simulink model "PID_nova_metoda"  (R2018a)
settings: Solver=ode4  StartTime=0.0  StopTime=100000.0  FixedStep=0.1  RelTol=1e-3
values from neighbouring files (symbols this model uses):
  Ca = pom1*10^-6    [projekat1.m]
  Cb = 10^-6    (= 1e-06)    [projekat1.m]
  Fa = 0.016667    [projekat1.m]
  Kp = mi*T*du/dy/tau    [projekat1.m]
  kw = 10^-14    (= 1e-14)    [projekat1.m]
  Td = T/8    [projekat1.m]
  Tf = Td/20    [projekat1.m]
  Ti = T    [projekat1.m]
  Tt = 0.01*Ti    (= 9.0009)    [projekat1.m]
  uep = eval (ue)    [projekat1.m]
  V = 30    [projekat1.m]
settings Model: Creator=Dusan Licina  LastModifiedBy=svorc

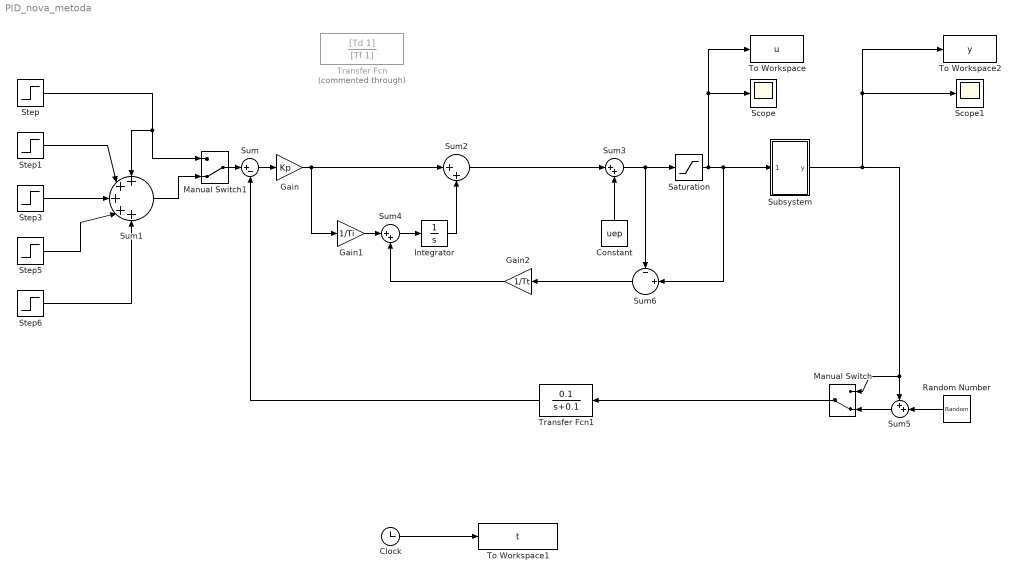
== system PID_nova_metoda ==
  Clock : Clock
  Constant : Constant  Value=uep
  Gain : Gain  Gain=Kp
  Gain1 : Gain  Gain=1/Ti
  Gain2 : Gain  Gain=1/Tt
  Integrator : Integrator
  Manual Switch : ManualSwitch  CurrentSetting=0
  Manual Switch1 : ManualSwitch  CurrentSetting=0
  Random Number : RandomNumber  Variance=0.1225  SampleTime=0.1
  Saturation : Saturate  UpperLimit=10*Fa  LowerLimit=0
  Scope : Scope
  Scope1 : Scope
  Step : Step  Time=0.1  After=7  SampleTime=0
  Step1 : Step  Time=10000  After=-0.5  SampleTime=0
  Step3 : Step  Time=30000  After=0.5  SampleTime=0
  Step5 : Step  Time=50000  After=0.5  SampleTime=0
  Step6 : Step  Time=70000  After=-0.5  SampleTime=0
  Subsystem : Subsystem
  Sum : Sum  Inputs=|+-
  Sum1 : Sum  Inputs=+|+|+|+|+
  Sum2 : Sum  Inputs=|++
  Sum3 : Sum  Inputs=|++
  Sum4 : Sum  Inputs=|++
  Sum5 : Sum  Inputs=++|
  Sum6 : Sum  Inputs=-|+||
  To Workspace : ToWorkspace  VariableName=u  SampleTime=-1
  To Workspace1 : ToWorkspace  VariableName=t  SampleTime=-1
  To Workspace2 : ToWorkspace  VariableName=y  SampleTime=-1
  Transfer Fcn : TransferFcn  Commented=through  Numerator=[Td 1]  Denominator=[Tf 1]
  Transfer Fcn1 : TransferFcn  Numerator=[0.1]  Denominator=[1 0.1]
  wires:
  Sum1/1 -> Manual Switch1/2
  Step1/1 -> Sum1/2
  Step/1 -> Manual Switch1/1, Sum1/1
  Sum/1 -> Gain/1
  Clock/1 -> To Workspace1/1
  Gain/1 -> Gain1/1, Sum2/1
  Manual Switch1/1 -> Sum/1
  Constant/1 -> Sum3/2
  Sum3/1 -> Saturation/1, Sum6/1
  Saturation/1 -> To Workspace/1, Scope/1, Sum6/2, Subsystem/1(Input)
  Sum5/1 -> Manual Switch/2
  Random Number/1 -> Sum5/2
  Subsystem/1(y) -> To Workspace2/1, Scope1/1, Manual Switch/1, Sum5/1
  Integrator/1 -> Sum2/2
  Gain1/1 -> Sum4/1
  Sum4/1 -> Integrator/1
  Sum6/1 -> Gain2/1
  Gain2/1 -> Sum4/2
  Manual Switch/1 -> Transfer Fcn1/1
  Transfer Fcn1/1 -> Sum/2
  Sum2/1 -> Sum3/1
  Step6/1 -> Sum1/5
  Step5/1 -> Sum1/4
  Step3/1 -> Sum1/3

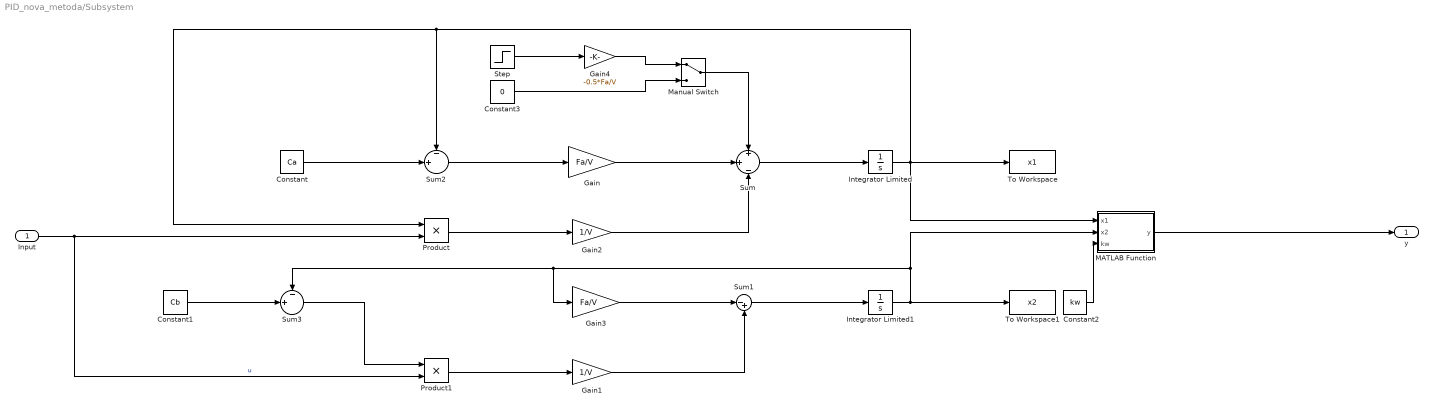
== system PID_nova_metoda/Subsystem ==
  Input : Inport
  Constant : Constant  Value=Ca
  Constant1 : Constant  Value=Cb
  Constant2 : Constant  Value=kw
  Constant3 : Constant  Value=0
  Gain : Gain  Gain=Fa/V
  Gain1 : Gain  Gain=1/V
  Gain2 : Gain  Gain=1/V
  Gain3 : Gain  Gain=Fa/V
  Gain4 : Gain  Gain=-0.5*Fa/V
  Integrator Limited : Integrator  LimitOutput=on  UpperSaturationLimit=Ca  LowerSaturationLimit=0
  Integrator Limited1 : Integrator  LimitOutput=on  UpperSaturationLimit=Cb  LowerSaturationLimit=0
  MATLAB Function : MATLAB Function  TreatAsAtomicUnit=on
  Manual Switch : ManualSwitch
  Product : Product
  Product1 : Product
  Step : Step  Time=80000  After=Ca  SampleTime=0
  Sum : Sum  Inputs=+|+|-
  Sum1 : Sum  Inputs=|-+
  Sum2 : Sum  Inputs=-|+||
  Sum3 : Sum  Inputs=-|+||
  To Workspace : ToWorkspace  VariableName=x1  SampleTime=-1
  To Workspace1 : ToWorkspace  VariableName=x2  SampleTime=-1
  y : Outport
  wires:
  Sum3/1 -> Product1/1
  Sum/1 -> Integrator Limited/1
  Gain/1 -> Sum/2
  Input/1 -> Product/2, Product1/2  "u"
  Gain3/1 -> Sum1/1
  Integrator Limited1/1 -> MATLAB Function/2(x2), Gain3/1, Sum3/1, To Workspace1/1
  Integrator Limited/1 -> To Workspace/1, MATLAB Function/1(x1), Sum2/1, Product/1
  Constant1/1 -> Sum3/2
  Sum1/1 -> Integrator Limited1/1
  Product1/1 -> Gain1/1
  Constant/1 -> Sum2/2
  MATLAB Function/1(y) -> y/1
  Gain1/1 -> Sum1/2
  Product/1 -> Gain2/1
  Sum2/1 -> Gain/1
  Constant2/1 -> MATLAB Function/3(kw)
  Gain2/1 -> Sum/3
  Step/1 -> Gain4/1
  Manual Switch/1 -> Sum/1
  Gain4/1 -> Manual Switch/1
  Constant3/1 -> Manual Switch/2

== matlab function PID_nova_metoda/Subsystem/MATLAB Function ==
  data: x1 input; y output; x2 input; kw input
function y = fcn(x1, x2, kw)

y = -log10(sqrt((x2-x1)^2 / 4 + kw) - (x2 - x1) / 2);
